simulink model "SG__MDL"  (R2022b)
settings: Solver=FixedStepAuto  StartTime=0.0  StopTime=Inf  FixedStep=ts  RelTol=1e-3  EnableMultiTasking=on
settings Model: SimulationMode=external  ExplicitPartitioning=on  DataflowThreadingImplementation=OpenMP  Creator=padlewsk  LastModifiedBy=padlewsk
settings SolverCC: ConcurrentTasks=on  AlgebraicLoopSolver=TrustRegion  PositivePriorityOrder=on  AutoInsertRateTranBlk=on
settings DataIOCC: SaveFormat=StructureWithTime
settings OptimizationCC: GainParamInheritBuiltInType=on  UseFloatMulNetSlope=on  RollThreshold=9  EfficientFloat2IntCast=on  SimCompilerOptimization=on
settings DebuggingCC: TasksWithSamePriorityMsg=none  UnconnectedInputMsg=warning  UnconnectedOutputMsg=warning  UnconnectedLineMsg=warning
settings HardwareCC: ProdBitPerLong=64  ProdLongLongMode=on  ProdHWDeviceType=Intel->x86-64 (Linux 64)
settings ModelReferenceCC: EnableRefExpFcnMdlSchedulingChecks=on
settings RTWCC: Description=Simulink Real-Time  SystemTargetFile=slrealtime.tlc  TemplateMakefile=slrealtime_default_tmf  Toolchain=Simulink Real-Time Toolchain  BuildConfiguration=Faster Runs  CodeExecutionProfiling=on  CodeProfilingInstrumentation=coarse  TargetLang=C++

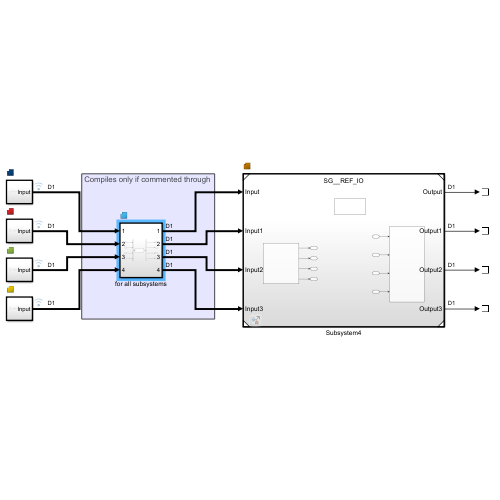
[thumbnail: Simulink's stored preview of the top-level diagram]
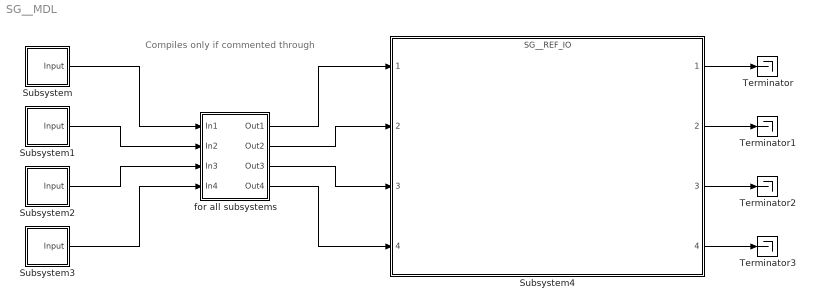
== system SG__MDL ==
  note: Compiles only if commented through
  Subsystem : Subsystem  TreatAsAtomicUnit=on
  Subsystem1 : Subsystem  TreatAsAtomicUnit=on
  Subsystem2 : Subsystem  TreatAsAtomicUnit=on
  Subsystem3 : Subsystem  TreatAsAtomicUnit=on
  Subsystem4 : ModelReference  ModelNameDialog=SG__REF_IO.slx  SimulationMode=Normal  ModelReferenceVersion=5.5
  Terminator{,1..3} (4 alike) : Terminator
  for all subsystems : Subsystem  TreatAsAtomicUnit=on
      settings: RTWSystemCode=Nonreusable function
  wires:
  Subsystem4/1 -> Terminator/1
  Subsystem4/2 -> Terminator1/1
  Subsystem4/3 -> Terminator2/1
  Subsystem4/4 -> Terminator3/1
  Subsystem/1(Input) -> for all subsystems/1(In1)
  Subsystem1/1(Input) -> for all subsystems/2(In2)
  Subsystem2/1(Input) -> for all subsystems/3(In3)
  Subsystem3/1(Input) -> for all subsystems/4(In4)
  for all subsystems/1(Out1) -> Subsystem4/1
  for all subsystems/2(Out2) -> Subsystem4/2
  for all subsystems/3(Out3) -> Subsystem4/3
  for all subsystems/4(Out4) -> Subsystem4/4

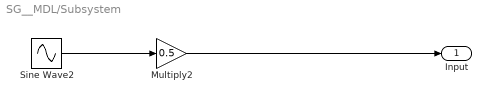
== system SG__MDL/Subsystem ==
  Multiply2 : Gain  Gain=0.5
  Sine Wave2 : Sin  Frequency=2*pi*10
  Input : Outport
  wires:
  Sine Wave2/1 -> Multiply2/1
  Multiply2/1 -> Input/1

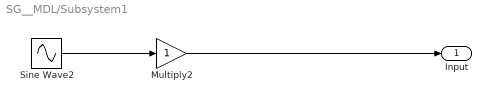
== system SG__MDL/Subsystem1 ==
  Multiply2 : Gain
  Sine Wave2 : Sin  Frequency=2*pi*10
  Input : Outport
  wires:
  Sine Wave2/1 -> Multiply2/1
  Multiply2/1 -> Input/1

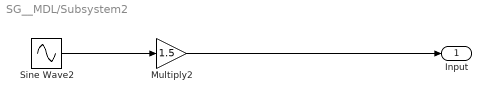
== system SG__MDL/Subsystem2 ==
  Multiply2 : Gain  Gain=1.5
  Sine Wave2 : Sin  Frequency=2*pi*10
  Input : Outport
  wires:
  Sine Wave2/1 -> Multiply2/1
  Multiply2/1 -> Input/1

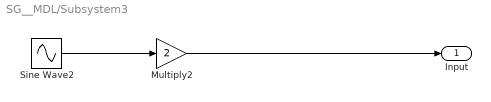
== system SG__MDL/Subsystem3 ==
  Multiply2 : Gain  Gain=2
  Sine Wave2 : Sin  Frequency=2*pi*10
  Input : Outport
  wires:
  Sine Wave2/1 -> Multiply2/1
  Multiply2/1 -> Input/1

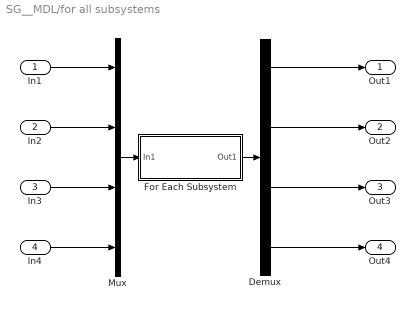
== system SG__MDL/for all subsystems ==
  In1 : Inport
  In2 : Inport  Port=2
  In3 : Inport  Port=3
  In4 : Inport  Port=4
  Demux : Demux
  For Each Subsystem : Subsystem  TreatAsAtomicUnit=on
  Mux : Mux
  Out1 : Outport
  Out2 : Outport  Port=2
  Out3 : Outport  Port=3
  Out4 : Outport  Port=4
  wires:
  For Each Subsystem/1(Out1) -> Demux/1
  In3/1 -> Mux/3
  Demux/2 -> Out2/1
  Mux/1 -> For Each Subsystem/1(In1)
  Demux/1 -> Out1/1
  In2/1 -> Mux/2
  In4/1 -> Mux/4
  In1/1 -> Mux/1
  Demux/3 -> Out3/1
  Demux/4 -> Out4/1

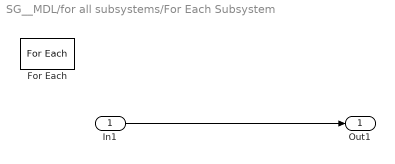
== system SG__MDL/for all subsystems/For Each Subsystem ==
  In1 : Inport  Partition=on  PartitionDimension=1  PartitionWidth=1  PartitionOffset=0
  For Each : ForEach  DisableCoverage=on
  Out1 : Outport  ConcatenationDimension=1
  wires:
  In1/1 -> Out1/1
